simulink model "BLDCmotorControl_FOC_R2017b_fixdt"  (R2017b)
settings: Solver=FixedStepDiscrete  StartTime=0  StopTime=0.5  FixedStep=Ts  MaxStep=1e-6  RelTol=1e-6  AbsTol=1e-6  EnableMultiTasking=on
PreLoadFcn:
  | addpath(pwd);
  | addpath(genpath('01_Libraries'));
  | addpath(genpath('02_Figures'));
  | addpath(genpath('03_CreateParamTable'));
InitFcn:
  | init_model;
values from neighbouring files (symbols this model uses):
  a_elecAngle = 60    [init_model.m]
  b_diagEna = 1    [init_model.m]
  b_fieldWeakEna = 0    [init_model.m]
  b_selPhaABCurrMeas = 1    [init_model.m]
  cf_currFilt = 0.12    [init_model.m]
  cf_idKb = 1000 * Ts_ctrl    (= 0.06)    [init_model.m]
  cf_idKi = 100 * Ts_ctrl    (= 0.006)    [init_model.m]
  cf_idKp = 1    [init_model.m]
  cf_iqKb = 1000 * Ts_ctrl    (= 0.06)    [init_model.m]
  cf_iqKi = 100 * Ts_ctrl    (= 0.006)    [init_model.m]
  cf_iqKiLimProt = 40.7 * Ts_ctrl    (= 0.002442)    [init_model.m]
  cf_iqKp = 0.5    [init_model.m]
  cf_iqKpLimProt = 7.2    [init_model.m]
  cf_nKb = 1000 * Ts_ctrl    (= 0.06)    [init_model.m]
  cf_nKi = 20.4 * Ts_ctrl    (= 0.001224)    [init_model.m]
  cf_nKp = 1.18    [init_model.m]
  cf_nKpLimProt = 5    [init_model.m]
  cf_speedCoef = round(f_ctrl * a_mechAngle * (pi/180) * (30/pi))    [init_model.m]
  CTRL_COM = 0    [init_model.m]
  dV_openRate = 1000 * Ts_ctrl    (= 0.06)    [init_model.m]
  dz_cntTrnsDetHi = 40    [init_model.m]
  dz_cntTrnsDetLo = 20    [init_model.m]
  i_max = i_max * i_sca    (= 750)    [init_model.m]
  id_fieldWeak_M1 = [  0   0  0.05  0.25    1    2    3    4  4.5  4.8   5   5] * i_sca    [init_model.m]
  iq_max_M1 = sqrt(i_max^2 - iq_max_XA.^2)    [init_model.m]
  n_commAcvLo = 15    [init_model.m]
  n_commDeacvHi = 30    [init_model.m]
  n_max = 800    [init_model.m]
  n_stdStillDet = 3    [init_model.m]
  OPEN_MODE = 0    [init_model.m]
  r_cos_M1 = cos((a_elecAngle_XA + 30)*(pi/180))    [init_model.m]
  r_errInpTgtThres = 200    [init_model.m]
  r_sin_M1 = sin((a_elecAngle_XA + 30)*(pi/180))    [init_model.m]
  r_whl = 6.5 * 2.54 * 1e-2 / 2    (= 0.08255)    [init_model.m]
  SPD_MODE = 2    [init_model.m]
  t_errDequal = 2.0 * f_ctrl    (= 32000)    [init_model.m]
  t_errQual = 0.6 * f_ctrl    (= 9600)    [init_model.m]
  TRQ_MODE = 3    [init_model.m]
  Ts = 5e-6    (= 5e-06)    [init_model.m]
  Ts_ctrl = 6e-5    (= 6e-05)    [init_model.m]
  Vd_max = 1000 - V_margin    (= 900)    [init_model.m]
  vec_hallToPos = [0 2 0 1 4 3 5 0]    [init_model.m]
  VLT_MODE = 1    [init_model.m]
  Vq_max_M1 = sqrt(Vd_max^2 - Vq_max_XA.^2)    [init_model.m]
  z_commutMap_M1 = [-1 -1  0  1  1  0 ... (first row only)    [init_model.m]
  z_ctrlModReq = 1    [init_model.m]
  z_ctrlTypSel = 1    [init_model.m]
  z_maxCntRst = 2000    [init_model.m]
undefined symbols (not defined in the file or in its folder): DiscIntNeverNeededParam, sigbuilder_block, V_max, V_min
libraries: BLDC_controller_Lib x11, simulink x11, powerlib x6, pePwmGenerator x1
(part 2 of 3)

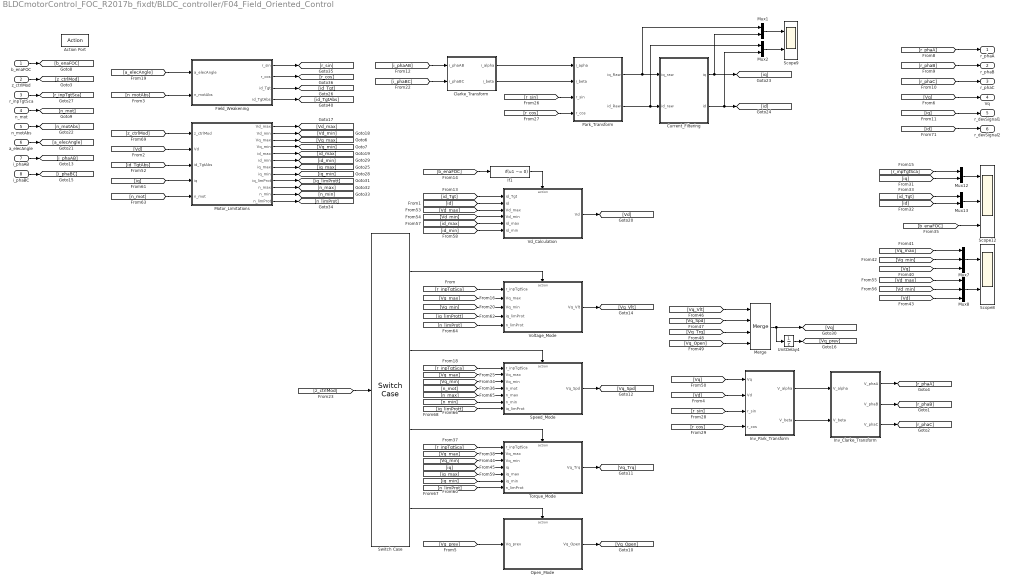
== system BLDCmotorControl_FOC_R2017b_fixdt/BLDC_controller/F04_Field_Oriented_Control ==
  b_enaFOC : Inport
  z_ctrlMod : Inport  Port=2
  r_inpTgtSca : Inport  Port=3
  n_mot : Inport  Port=4
  n_motAbs : Inport  Port=5
  a_elecAngle : Inport  Port=6
  i_phaAB : Inport  Port=7
  i_phaBC : Inport  Port=8
  Action Port : ActionPort  InitializeStates=reset  ActionType=then
  Clarke_Transform : Subsystem
  Current_Filtering : Subsystem
  Field_Weakening : Subsystem
  If1 : If  IfExpression=u1 ~= 0  ShowElse=off
  Inv_Clarke_Transform : Subsystem
  Inv_Park_Transform : Subsystem
  Merge : Merge  Inputs=4
  Motor_Limitations : Subsystem
  Mux{1..2,12..13} (4 alike) : Mux  Inputs=2
  Mux7 : Mux  Inputs=3
  Mux8 : Mux  Inputs=3
  Open_Mode : Subsystem
  Park_Transform : Subsystem
  Scope12 : Scope  NumInputPorts=3
  Scope8 : Scope  NumInputPorts=2
  Scope9 : Scope  NumInputPorts=2
  Speed_Mode : Subsystem
  Switch Case : SwitchCase  CaseConditions={VLT_MODE, SPD_MODE, TRQ_MODE}
  Torque_Mode : Subsystem
  UnitDelay4 : UnitDelay  SampleTime=-1
      settings: AttributesFormatString=Ini=%<X0>
  Vd_Calculation : Subsystem
  Voltage_Mode : Subsystem
  r_phaA : Outport  OutputWhenDisabled=reset  InitialOutput=0
  r_phaB : Outport  Port=2  OutputWhenDisabled=reset  InitialOutput=0
  "r_phaC " : Outport  Port=3  OutputWhenDisabled=reset  InitialOutput=0
  Vq : Outport  Port=4  OutputWhenDisabled=reset  InitialOutput=0
  r_devSignal1 : Outport  Port=5  OutputWhenDisabled=reset  InitialOutput=0
  r_devSignal2 : Outport  Port=6  OutputWhenDisabled=reset  InitialOutput=0
  wires:
  [r_phaA] -> r_phaA/1
  [r_phaB] -> r_phaB/1
  [r_phaC] -> "r_phaC "/1
  Inv_Park_Transform/1(V_alpha) -> Inv_Clarke_Transform/1(V_alpha)
  Inv_Park_Transform/2(V_beta) -> Inv_Clarke_Transform/2(V_beta)
  i_phaAB/1 -> [i_phaAB]
  i_phaBC/1 -> [i_phaBC]
  Inv_Clarke_Transform/1(V_phaA) -> [r_phaA]
  Inv_Clarke_Transform/2(V_phaB) -> [r_phaB]
  Inv_Clarke_Transform/3(V_phaC) -> [r_phaC]
  Clarke_Transform/1(i_alpha) -> Park_Transform/1(i_apha)
  Clarke_Transform/2(i_beta) -> Park_Transform/2(i_beta)
  Mux12/1 -> Scope12/1
  Mux13/1 -> Scope12/2
  [r_sin] -> Park_Transform/3(r_sin)
  [r_cos] -> Park_Transform/4(r_cos)
  [r_sin] -> Inv_Park_Transform/3(r_sin)
  [r_cos] -> Inv_Park_Transform/4(r_cos)
  [r_inpTgtSca] -> Mux12/1
  [iq] -> Mux12/2
  [id] -> Mux13/2
  [id_Tgt] -> Mux13/1
  r_inpTgtSca/1 -> [r_inpTgtSca]
  [i_phaAB] -> Clarke_Transform/1(i_phaAB)
  [i_phaBC] -> Clarke_Transform/2(i_phaBC)
  [Vd_max] -> Mux8/1
  [Vd] -> Mux8/3
  Mux8/1 -> Scope8/2
  [Vd_min] -> Mux8/2
  [Vq] -> Mux7/3
  Mux7/1 -> Scope8/1
  [Vq_max] -> Mux7/1
  [Vq_min] -> Mux7/2
  Park_Transform/2(id_Raw) -> Current_Filtering/2(id_raw), Mux2/1
  Park_Transform/1(iq_Raw) -> Current_Filtering/1(iq_raw), Mux1/1
  Current_Filtering/1(iq) -> [iq], Mux1/2
  Current_Filtering/2(id) -> [id], Mux2/2
  [Vq] -> Vq/1
  [id] -> Vd_Calculation/2(id)
  [id_Tgt] -> Vd_Calculation/1(id_Tgt)
  b_enaFOC/1 -> [b_enaFOC]
  If1/1 -> Vd_Calculation/Action
  [b_enaFOC] -> If1/1
  [Vd] -> Inv_Park_Transform/2(Vd)
  z_ctrlMod/1 -> [z_ctrlMod]
  n_mot/1 -> [n_mot]
  [b_enaFOC] -> Scope12/3
  [z_ctrlMod] -> Switch Case/1
  [Vq_prev] -> Open_Mode/1(Vq_prev)
  Open_Mode/1(Vq_Open) -> [Vq_Open]
  Torque_Mode/1(Vq_Trq) -> [Vq_Trq]
  Speed_Mode/1(Vq_Spd) -> [Vq_Spd]
  Voltage_Mode/1(Vq_Vlt) -> [Vq_Vlt]
  [r_inpTgtSca] -> Voltage_Mode/1(r_inpTgtSca)
  [Vq_max] -> Voltage_Mode/2(Vq_max)
  [Vq_min] -> Voltage_Mode/3(Vq_min)
  [r_inpTgtSca] -> Speed_Mode/1(r_inpTgtSca)
  [Vq_max] -> Speed_Mode/2(Vq_max)
  [Vq_min] -> Speed_Mode/3(Vq_min)
  [n_mot] -> Speed_Mode/4(n_mot)
  [Vq_min] -> Torque_Mode/3(Vq_min)
  [Vq_max] -> Torque_Mode/2(Vq_max)
  [r_inpTgtSca] -> Torque_Mode/1(r_inpTgtSca)
  [iq] -> Torque_Mode/4(iq)
  Switch Case/1 -> Voltage_Mode/Action
  Switch Case/2 -> Speed_Mode/Action
  Switch Case/3 -> Torque_Mode/Action
  Switch Case/4 -> Open_Mode/Action
  [Vq_Vlt] -> Merge/1
  [Vq_Spd] -> Merge/2
  [Vq_Trq] -> Merge/3
  [Vq_Open] -> Merge/4
  [Vq] -> Inv_Park_Transform/1(Vq)
  Merge/1 -> UnitDelay4/1, [Vq]
  UnitDelay4/1 -> [Vq_prev]
  Motor_Limitations/3(Vq_max) -> [Vq_max]
  Motor_Limitations/4(Vq_min) -> [Vq_min]
  [Vd] -> Motor_Limitations/2(Vd)
  [id_TgtAbs] -> Motor_Limitations/3(id_TgtAbs)
  Motor_Limitations/2(Vd_min) -> [Vd_min]
  Motor_Limitations/1(Vd_max) -> [Vd_max]
  [Vd_max] -> Vd_Calculation/3(Vd_max)
  [Vd_min] -> Vd_Calculation/4(Vd_min)
  Motor_Limitations/5(id_max) -> [id_max]
  Motor_Limitations/6(id_min) -> [id_min]
  Motor_Limitations/7(iq_max) -> [iq_max]
  Motor_Limitations/8(iq_min) -> [iq_min]
  [id_max] -> Vd_Calculation/5(id_max)
  [id_min] -> Vd_Calculation/6(id_min)
  [iq_max] -> Torque_Mode/5(iq_max)
  [iq_min] -> Torque_Mode/6(iq_min)
  [iq] -> Motor_Limitations/4(iq)
  Motor_Limitations/9(iq_limProt) -> [iq_limPrott]
  [iq_limPrott] -> Voltage_Mode/4(iq_limProt)
  Motor_Limitations/11(n_min) -> [n_min]
  Motor_Limitations/10(n_max) -> [n_max]
  Motor_Limitations/12(n_limProt) -> [n_limProt]
  [n_mot] -> Motor_Limitations/5(n_mot)
  [n_limProt] -> Voltage_Mode/5(n_limProt)
  [n_max] -> Speed_Mode/5(n_max)
  [n_min] -> Speed_Mode/6(n_min)
  [n_limProt] -> Torque_Mode/7(n_limProt)
  [iq_limPrott] -> Speed_Mode/7(iq_limProt)
  [z_ctrlMod] -> Motor_Limitations/1(z_ctrlMod)
  n_motAbs/1 -> [n_motAbs]
  Field_Weakening/1(r_sin) -> [r_sin]
  Field_Weakening/2(r_cos) -> [r_cos]
  [a_elecAngle] -> Field_Weakening/1(a_elecAngle)
  Field_Weakening/3(id_Tgt) -> [id_Tgt]
  [n_motAbs] -> Field_Weakening/2(n_motAbs)
  a_elecAngle/1 -> [a_elecAngle]
  Mux1/1 -> Scope9/1
  Mux2/1 -> Scope9/2
  [id] -> r_devSignal2/1
  [iq] -> r_devSignal1/1
  Field_Weakening/4(id_TgtAbs) -> [id_TgtAbs]
  Vd_Calculation/1(Vd) -> [Vd]

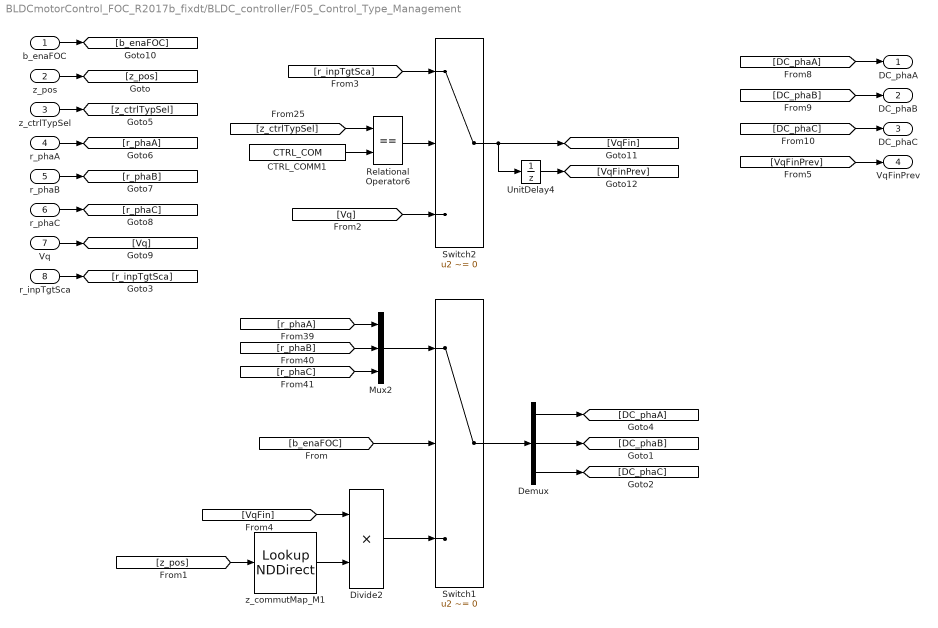
== system BLDCmotorControl_FOC_R2017b_fixdt/BLDC_controller/F05_Control_Type_Management ==
  b_enaFOC : Inport
  z_pos : Inport  Port=2
  z_ctrlTypSel : Inport  Port=3
  r_phaA : Inport  Port=4
  r_phaB : Inport  Port=5
  r_phaC : Inport  Port=6
  Vq : Inport  Port=7
  r_inpTgtSca : Inport  Port=8
  CTRL_COMM1 : Constant  Value=CTRL_COM  OutDataTypeStr=Inherit: Inherit via back propagation
  Demux : Demux  Outputs=3
  Divide2 : Product  Inputs=**  RndMeth=Simplest  OutDataTypeStr=Inherit: Same as first input
  Mux2 : Mux  Inputs=3
  Relational Operator6 : RelationalOperator  Operator===  OutDataTypeStr=boolean  RndMeth=Simplest
  Switch1 : Switch  Criteria=u2 ~= 0  OutDataTypeStr=Inherit: Inherit via back propagation  RndMeth=Zero
  Switch2 : Switch  Criteria=u2 ~= 0  OutDataTypeStr=Inherit: Inherit via back propagation  RndMeth=Zero
  UnitDelay4 : UnitDelay  SampleTime=-1
      settings: AttributesFormatString=Ini=%<X0>
  z_commutMap_M1 : LookupNDDirect  InputsSelectThisObjectFromTable=Column  Table=z_commutMap_M1  DiagnosticForOutOfRangeInput=None  TableDataTypeStr=int16
  DC_phaA : Outport  OutputWhenDisabled=reset  InitialOutput=0
  DC_phaB : Outport  Port=2  OutputWhenDisabled=reset  InitialOutput=0
  "DC_phaC " : Outport  Port=3  OutputWhenDisabled=reset  InitialOutput=0
  VqFinPrev : Outport  Port=4  OutputWhenDisabled=reset  InitialOutput=0
  wires:
  Demux/3 -> [DC_phaC]
  Demux/2 -> [DC_phaB]
  Demux/1 -> [DC_phaA]
  z_pos/1 -> [z_pos]
  [DC_phaC] -> "DC_phaC "/1
  [DC_phaB] -> DC_phaB/1
  [DC_phaA] -> DC_phaA/1
  [z_pos] -> z_commutMap_M1/1
  Switch1/1 -> Demux/1
  r_phaA/1 -> [r_phaA]
  r_phaB/1 -> [r_phaB]
  r_phaC/1 -> [r_phaC]
  Vq/1 -> [Vq]
  [r_phaA] -> Mux2/1
  [r_phaB] -> Mux2/2
  [r_phaC] -> Mux2/3
  z_commutMap_M1/1 -> Divide2/2
  Divide2/1 -> Switch1/3
  b_enaFOC/1 -> [b_enaFOC]
  Mux2/1 -> Switch1/1
  [b_enaFOC] -> Switch1/2
  [z_ctrlTypSel] -> Relational Operator6/1
  CTRL_COMM1/1 -> Relational Operator6/2
  Relational Operator6/1 -> Switch2/2
  r_inpTgtSca/1 -> [r_inpTgtSca]
  [Vq] -> Switch2/3
  z_ctrlTypSel/1 -> [z_ctrlTypSel]
  Switch2/1 -> UnitDelay4/1, [VqFin]
  UnitDelay4/1 -> [VqFinPrev]
  [VqFin] -> Divide2/1
  [VqFinPrev] -> VqFinPrev/1
  [r_inpTgtSca] -> Switch2/1

== system BLDCmotorControl_FOC_R2017b_fixdt/BLDC_controller/Implemented_control_methods ==

== system BLDCmotorControl_FOC_R2017b_fixdt/BLDC_model_closed/__InputSSForSFun__ ==
  gates_PWM : Inport
  Tm_Nm : Inport  Port=2
  __UniqueOutportName__1__ : Outport
  __UniqueOutportName__2__ : Outport  Port=2
  wires:
  gates_PWM/1 -> __UniqueOutportName__1__/1
  Tm_Nm/1 -> __UniqueOutportName__2__/1

== system BLDCmotorControl_FOC_R2017b_fixdt/BLDC_model_closed/__OutputSSForSFun__ ==
  __UniqueInportName__1__ : Inport
  __UniqueInportName__2__ : Inport  Port=2
  __UniqueInportName__3__ : Inport  Port=3
  __UniqueInportName__4__ : Inport  Port=4
  __UniqueInportName__5__ : Inport  Port=5
  __UniqueInportName__6__ : Inport  Port=6
  __UniqueInportName__7__ : Inport  Port=7
  __UniqueInportName__8__ : Inport  Port=8
  __UniqueInportName__9__ : Inport  Port=9
  __UniqueInportName__10__ : Inport  Port=10
  __UniqueInportName__11__ : Inport  Port=11
  __UniqueInportName__12__ : Inport  Port=12
  Mux1 : BusCreator  Inputs=12
  motor_out : Outport
  wires:
  __UniqueInportName__1__/1 -> Mux1/1  "Stator current is_a (A)"
  __UniqueInportName__2__/1 -> Mux1/2  "Stator current is_b (A)"
  __UniqueInportName__3__/1 -> Mux1/3  "Stator current is_c (A)"
  __UniqueInportName__4__/1 -> Mux1/4  "Stator back EMF e_a (V)"
  __UniqueInportName__5__/1 -> Mux1/5  "Stator back EMF e_b (V)"
  __UniqueInportName__6__/1 -> Mux1/6  "Stator back EMF e_cV)"
  __UniqueInportName__7__/1 -> Mux1/7  "Hall effect signal h_a"
  __UniqueInportName__8__/1 -> Mux1/8  "Hall effect signal h_b"
  __UniqueInportName__9__/1 -> Mux1/9  "Hall effect signal h_c"
  __UniqueInportName__10__/1 -> Mux1/10  "Rotor speed wm (rad/s)"
  __UniqueInportName__11__/1 -> Mux1/11  "Rotor angle thetam (rad)"
  __UniqueInportName__12__/1 -> Mux1/12  "Electromagnetic torque Te (N*m)"
  Mux1/1 -> motor_out/1

== system BLDCmotorControl_FOC_R2017b_fixdt/PWM_gates/PWM_generator1 ==
  DC : Inport  SampleTime=Ts
  PWM_generator_sfcn : S-Function  FunctionName=PWM_generator_sf  SFunctionModules=""  SFunctionDeploymentMode=off  EnableBusSupport=off  SFcnStateName=DWORK0  mask{rtw_sf_name=PWM_generator_sf, showVar=off}
      mask prompts: rtw_sf_name "Simulink:masks:GenSFuncName_MP"; showVar "Simulink:masks:GenSFuncShowModuleList_MP"
      mask help: Simulink:masks:GenSFuncDesc_MD
      mask init: same as BLDCmotorControl_FOC_R2017b_fixdt/BLDC_model_closed/BLDC_model_sfcn
      settings: SFcnIsStateOwnerBlock=on
      settings: CopyFcn=|
      | if ~strcmp(get_param(gcb,'Linkstatus'),'none') && ...
      | ~strcmp(get_param(gcb,'Linkstatus'),'implicit')
      |   set_param(gcb,'LinkStatus','none');
      | end
      mask Help: eval('feval(''rtwprivate'',''rtwhelpview'',''rtw_sfcn_block'')');
      mask Display:
      | port_label('input',1,'DC');
      | port_label('output',1,'PWM');
  __InputSSForSFun__ : Subsystem
  __OutputSSForSFun__ : Subsystem
  PWM : Outport
  wires:
  __OutputSSForSFun__/1(PWM) -> PWM/1
  PWM_generator_sfcn/1 -> __OutputSSForSFun__/1(__UniqueInportName__1__)
  __InputSSForSFun__/1(__UniqueOutportName__1__) -> PWM_generator_sfcn/1
  DC/1 -> __InputSSForSFun__/1(DC)

== system BLDCmotorControl_FOC_R2017b_fixdt/PWM_gates/PWM_generator12 ==
  DC : Inport  SampleTime=Ts
  PWM_generator_sfcn : S-Function  FunctionName=PWM_generator_sf  SFunctionModules=""  SFunctionDeploymentMode=off  EnableBusSupport=off  SFcnStateName=DWORK0  mask{rtw_sf_name=PWM_generator_sf, showVar=off}
      mask prompts: rtw_sf_name "Simulink:masks:GenSFuncName_MP"; showVar "Simulink:masks:GenSFuncShowModuleList_MP"
      mask help: Simulink:masks:GenSFuncDesc_MD
      mask init: same as BLDCmotorControl_FOC_R2017b_fixdt/BLDC_model_closed/BLDC_model_sfcn
      settings: SFcnIsStateOwnerBlock=on
      settings: CopyFcn=|
      | if ~strcmp(get_param(gcb,'Linkstatus'),'none') && ...
      | ~strcmp(get_param(gcb,'Linkstatus'),'implicit')
      |   set_param(gcb,'LinkStatus','none');
      | end
      mask Help: eval('feval(''rtwprivate'',''rtwhelpview'',''rtw_sfcn_block'')');
      mask Display:
      | port_label('input',1,'DC');
      | port_label('output',1,'PWM');
  __InputSSForSFun__ : Subsystem
  __OutputSSForSFun__ : Subsystem
  PWM : Outport
  wires:
  DC/1 -> __InputSSForSFun__/1(DC)
  __InputSSForSFun__/1(__UniqueOutportName__1__) -> PWM_generator_sfcn/1
  PWM_generator_sfcn/1 -> __OutputSSForSFun__/1(__UniqueInportName__1__)
  __OutputSSForSFun__/1(PWM) -> PWM/1

== system BLDCmotorControl_FOC_R2017b_fixdt/PWM_gates/PWM_generator2 ==
  DC : Inport  SampleTime=Ts
  PWM_generator_sfcn : S-Function  FunctionName=PWM_generator_sf  SFunctionModules=""  SFunctionDeploymentMode=off  EnableBusSupport=off  SFcnStateName=DWORK0  mask{rtw_sf_name=PWM_generator_sf, showVar=off}
      mask prompts: rtw_sf_name "Simulink:masks:GenSFuncName_MP"; showVar "Simulink:masks:GenSFuncShowModuleList_MP"
      mask help: Simulink:masks:GenSFuncDesc_MD
      mask init: same as BLDCmotorControl_FOC_R2017b_fixdt/BLDC_model_closed/BLDC_model_sfcn
      settings: SFcnIsStateOwnerBlock=on
      settings: CopyFcn=|
      | if ~strcmp(get_param(gcb,'Linkstatus'),'none') && ...
      | ~strcmp(get_param(gcb,'Linkstatus'),'implicit')
      |   set_param(gcb,'LinkStatus','none');
      | end
      mask Help: eval('feval(''rtwprivate'',''rtwhelpview'',''rtw_sfcn_block'')');
      mask Display:
      | port_label('input',1,'DC');
      | port_label('output',1,'PWM');
  __InputSSForSFun__ : Subsystem
  __OutputSSForSFun__ : Subsystem
  PWM : Outport
  wires:
  DC/1 -> __InputSSForSFun__/1(DC)
  __InputSSForSFun__/1(__UniqueOutportName__1__) -> PWM_generator_sfcn/1
  PWM_generator_sfcn/1 -> __OutputSSForSFun__/1(__UniqueInportName__1__)
  __OutputSSForSFun__/1(PWM) -> PWM/1

== system BLDCmotorControl_FOC_R2017b_fixdt/PWM_gates/PWM_generator3 ==
  DC : Inport  SampleTime=Ts
  PWM_generator_sfcn : S-Function  FunctionName=PWM_generator_sf  SFunctionModules=""  SFunctionDeploymentMode=off  EnableBusSupport=off  SFcnStateName=DWORK0  mask{rtw_sf_name=PWM_generator_sf, showVar=off}
      mask prompts: rtw_sf_name "Simulink:masks:GenSFuncName_MP"; showVar "Simulink:masks:GenSFuncShowModuleList_MP"
      mask help: Simulink:masks:GenSFuncDesc_MD
      mask init: same as BLDCmotorControl_FOC_R2017b_fixdt/BLDC_model_closed/BLDC_model_sfcn
      settings: SFcnIsStateOwnerBlock=on
      settings: CopyFcn=|
      | if ~strcmp(get_param(gcb,'Linkstatus'),'none') && ...
      | ~strcmp(get_param(gcb,'Linkstatus'),'implicit')
      |   set_param(gcb,'LinkStatus','none');
      | end
      mask Help: eval('feval(''rtwprivate'',''rtwhelpview'',''rtw_sfcn_block'')');
      mask Display:
      | port_label('input',1,'DC');
      | port_label('output',1,'PWM');
  __InputSSForSFun__ : Subsystem
  __OutputSSForSFun__ : Subsystem
  PWM : Outport
  wires:
  __OutputSSForSFun__/1(PWM) -> PWM/1
  PWM_generator_sfcn/1 -> __OutputSSForSFun__/1(__UniqueInportName__1__)
  __InputSSForSFun__/1(__UniqueOutportName__1__) -> PWM_generator_sfcn/1
  DC/1 -> __InputSSForSFun__/1(DC)

== system BLDCmotorControl_FOC_R2017b_fixdt/PWM_gates/PWM_generator4 ==
  DC : Inport  SampleTime=Ts
  PWM_generator_sfcn : S-Function  FunctionName=PWM_generator_sf  SFunctionModules=""  SFunctionDeploymentMode=off  EnableBusSupport=off  SFcnStateName=DWORK0  mask{rtw_sf_name=PWM_generator_sf, showVar=off}
      mask prompts: rtw_sf_name "Simulink:masks:GenSFuncName_MP"; showVar "Simulink:masks:GenSFuncShowModuleList_MP"
      mask help: Simulink:masks:GenSFuncDesc_MD
      mask init: same as BLDCmotorControl_FOC_R2017b_fixdt/BLDC_model_closed/BLDC_model_sfcn
      settings: SFcnIsStateOwnerBlock=on
      settings: CopyFcn=|
      | if ~strcmp(get_param(gcb,'Linkstatus'),'none') && ...
      | ~strcmp(get_param(gcb,'Linkstatus'),'implicit')
      |   set_param(gcb,'LinkStatus','none');
      | end
      mask Help: eval('feval(''rtwprivate'',''rtwhelpview'',''rtw_sfcn_block'')');
      mask Display:
      | port_label('input',1,'DC');
      | port_label('output',1,'PWM');
  __InputSSForSFun__ : Subsystem
  __OutputSSForSFun__ : Subsystem
  PWM : Outport
  wires:
  DC/1 -> __InputSSForSFun__/1(DC)
  __InputSSForSFun__/1(__UniqueOutportName__1__) -> PWM_generator_sfcn/1
  PWM_generator_sfcn/1 -> __OutputSSForSFun__/1(__UniqueInportName__1__)
  __OutputSSForSFun__/1(PWM) -> PWM/1

== system BLDCmotorControl_FOC_R2017b_fixdt/PWM_gates/PWM_generator5 ==
  DC : Inport  SampleTime=Ts
  PWM_generator_sfcn : S-Function  FunctionName=PWM_generator_sf  SFunctionModules=""  SFunctionDeploymentMode=off  EnableBusSupport=off  SFcnStateName=DWORK0  mask{rtw_sf_name=PWM_generator_sf, showVar=off}
      mask prompts: rtw_sf_name "Simulink:masks:GenSFuncName_MP"; showVar "Simulink:masks:GenSFuncShowModuleList_MP"
      mask help: Simulink:masks:GenSFuncDesc_MD
      mask init: same as BLDCmotorControl_FOC_R2017b_fixdt/BLDC_model_closed/BLDC_model_sfcn
      settings: SFcnIsStateOwnerBlock=on
      settings: CopyFcn=|
      | if ~strcmp(get_param(gcb,'Linkstatus'),'none') && ...
      | ~strcmp(get_param(gcb,'Linkstatus'),'implicit')
      |   set_param(gcb,'LinkStatus','none');
      | end
      mask Help: eval('feval(''rtwprivate'',''rtwhelpview'',''rtw_sfcn_block'')');
      mask Display:
      | port_label('input',1,'DC');
      | port_label('output',1,'PWM');
  __InputSSForSFun__ : Subsystem
  __OutputSSForSFun__ : Subsystem
  PWM : Outport
  wires:
  __OutputSSForSFun__/1(PWM) -> PWM/1
  PWM_generator_sfcn/1 -> __OutputSSForSFun__/1(__UniqueInportName__1__)
  __InputSSForSFun__/1(__UniqueOutportName__1__) -> PWM_generator_sfcn/1
  DC/1 -> __InputSSForSFun__/1(DC)

== system BLDCmotorControl_FOC_R2017b_fixdt/PWM_gates/signal_log6 ==
  PWM : Inport
  Terminator_1 : Terminator
  wires:
  PWM/1 -> Terminator_1/1  "PWM"

== system BLDCmotorControl_FOC_R2017b_fixdt/filtLowPass/Low_Pass_Filter1 ==
  u : Inport
  coef : Inport  Port=2
  Constant1 : Constant  OutDataTypeStr=Inherit: Inherit via back propagation
  Divide1 : Product  Inputs=**  RndMeth=Simplest  OutDataTypeStr=Inherit: Same as first input
  Divide2 : Product  Inputs=**  RndMeth=Simplest  OutDataTypeStr=Inherit: Same as first input
  Sum1 : Sum  OutDataTypeStr=fixdt(1,16,4)  RndMeth=Simplest  SaturateOnIntegerOverflow=on  InputSameDT=on
  Sum5 : Sum  Inputs=+-  RndMeth=Simplest  InputSameDT=on  OutDataTypeStr=Inherit: Same as first input
  UnitDelay3 : UnitDelay  SampleTime=-1
  y : Outport
  wires:
  u/1 -> Divide1/1
  Sum1/1 -> UnitDelay3/1, y/1
  Constant1/1 -> Sum5/1
  Divide2/1 -> Sum1/2
  UnitDelay3/1 -> Divide2/1
  Sum5/1 -> Divide2/2
  coef/1 -> Sum5/2, Divide1/2
  Divide1/1 -> Sum1/1

== system BLDCmotorControl_FOC_R2017b_fixdt/BLDC_controller/F01_Estimations/F01_01_Input_Scaling ==
  note: Input Scaling [-1000,1000] → [min,max]
  z_ctrlTypSel : Inport
  r_inpTgt : Inport  Port=2
  z_ctrlModPrev : Inport  Port=3
  Commutation_Control_Type : Subsystem
  FOC_Control_Type : Subsystem
  If1 : If  IfExpression=u1 == CTRL_COM
  Merge : Merge
  r_inpTgtSca : Outport  OutputWhenDisabled=reset  InitialOutput=0
  wires:
  Commutation_Control_Type/1(r_inpTgtScaCOM) -> Merge/1
  [r_inpTgt] -> FOC_Control_Type/1(r_inpTgt)
  [r_inpTgtSca] -> r_inpTgtSca/1
  If1/1 -> Commutation_Control_Type/Action
  z_ctrlTypSel/1 -> [z_ctrlTypSel]
  [z_ctrlTypSel] -> If1/1
  FOC_Control_Type/1(r_inpTgtScaFOC) -> Merge/2
  [r_inpTgt] -> Commutation_Control_Type/1(r_inpTgt)
  r_inpTgt/1 -> [r_inpTgt]
  Merge/1 -> [r_inpTgtSca]
  If1/2 -> FOC_Control_Type/Action
  [z_ctrlModPrev] -> FOC_Control_Type/2(z_ctrlModPrev)
  z_ctrlModPrev/1 -> [z_ctrlModPrev]

== system BLDCmotorControl_FOC_R2017b_fixdt/BLDC_controller/F01_Estimations/F01_02_Edge_Detector ==
  b_hallA : Inport
  b_hallB : Inport  Port=2
  b_hallC : Inport  Port=3
  Logical Operator : Logic  Operator=XOR  Inputs=6  AllPortsSameDT=off  OutDataTypeStr=boolean
  UnitDelay1 : UnitDelay  SampleTime=-1
      settings: AttributesFormatString=Ini=%<X0>
  UnitDelay2 : UnitDelay  SampleTime=-1
      settings: AttributesFormatString=Ini=%<X0>
  UnitDelay3 : UnitDelay  SampleTime=-1
      settings: AttributesFormatString=Ini=%<X0>
  "b_edge " : Outport  OutputWhenDisabled=reset  InitialOutput=0
  wires:
  b_hallA/1 -> Logical Operator/1, UnitDelay3/1
  b_hallC/1 -> Logical Operator/3, UnitDelay2/1
  b_hallB/1 -> Logical Operator/2, UnitDelay1/1
  UnitDelay1/1 -> Logical Operator/5
  UnitDelay2/1 -> Logical Operator/6
  UnitDelay3/1 -> Logical Operator/4
  Logical Operator/1 -> "b_edge "/1

== system BLDCmotorControl_FOC_R2017b_fixdt/BLDC_controller/F01_Estimations/F01_03_Position_Calculation ==
  note: This calculates the low resolution position based on Hall sensors.
  b_hallA : Inport
  b_hallB : Inport  Port=2
  b_hallC : Inport  Port=3
  Selector : Selector  IndexMode=Zero-based  InputPortWidth=length(vec_hallToPos)  IndexOptions=Index vector (port)  Indices=[1 3]  OutputSizes=1
  Sum : Sum  Inputs=+++  RndMeth=Simplest  OutDataTypeStr=Inherit: Same as first input
  g_Ha : Gain  Gain=4  OutDataTypeStr=Inherit: Inherit via back propagation  RndMeth=Zero  ParamDataTypeStr=Inherit: Same as input
  g_Hb : Gain  Gain=2  OutDataTypeStr=Inherit: Inherit via back propagation  RndMeth=Simplest  ParamDataTypeStr=Inherit: Same as input
  vec_hallToPos : Constant  Value=vec_hallToPos  OutDataTypeStr=int8
  z_posRaw : Outport  OutputWhenDisabled=reset  InitialOutput=0
  "z_pos " : Outport  Port=2  OutputWhenDisabled=reset  InitialOutput=0
  wires:
  b_hallC/1 -> Sum/3
  g_Ha/1 -> Sum/1
  g_Hb/1 -> Sum/2
  Sum/1 -> z_posRaw/1, Selector/2
  b_hallA/1 -> g_Ha/1
  b_hallB/1 -> g_Hb/1
  vec_hallToPos/1 -> Selector/1
  Selector/1 -> "z_pos "/1

== system BLDCmotorControl_FOC_R2017b_fixdt/BLDC_controller/F01_Estimations/F01_04_Direction_Detection ==
  z_pos : Inport
  Action Port : ActionPort  ActionType=then
  Constant20 : Constant  Value=-5  OutDataTypeStr=Inherit: Inherit via back propagation
  Constant23 : Constant  Value=-1  OutDataTypeStr=int8
  Constant24 : Constant  OutDataTypeStr=int8
  Constant8 : Constant  OutDataTypeStr=Inherit: Inherit via back propagation
  Logical Operator3 : Logic  Operator=OR  AllPortsSameDT=off  OutDataTypeStr=boolean
  Relational Operator1 : RelationalOperator  Operator===  OutDataTypeStr=boolean  RndMeth=Simplest
  Relational Operator6 : RelationalOperator  Operator===  OutDataTypeStr=boolean  RndMeth=Simplest
  Sum2 : Sum  Inputs=|+-  RndMeth=Zero  InputSameDT=on  OutDataTypeStr=Inherit: Same as first input
  Switch2 : Switch  Criteria=u2 ~= 0  OutDataTypeStr=Inherit: Inherit via back propagation  RndMeth=Simplest
  UnitDelay2 : UnitDelay  SampleTime=-1
  UnitDelay3 : UnitDelay  SampleTime=-1
      settings: AttributesFormatString=Ini=%<X0>
  z_dir : Outport
  z_dirPrev : Outport  Port=2
  wires:
  UnitDelay2/1 -> Sum2/2
  Relational Operator1/1 -> Logical Operator3/1
  Constant8/1 -> Relational Operator1/2
  Sum2/1 -> Relational Operator6/1, Relational Operator1/1
  Relational Operator6/1 -> Logical Operator3/2
  Constant20/1 -> Relational Operator6/2
  Constant24/1 -> Switch2/1
  Constant23/1 -> Switch2/3
  Logical Operator3/1 -> Switch2/2
  z_pos/1 -> Sum2/1, UnitDelay2/1
  Switch2/1 -> UnitDelay3/1, z_dir/1
  UnitDelay3/1 -> z_dirPrev/1

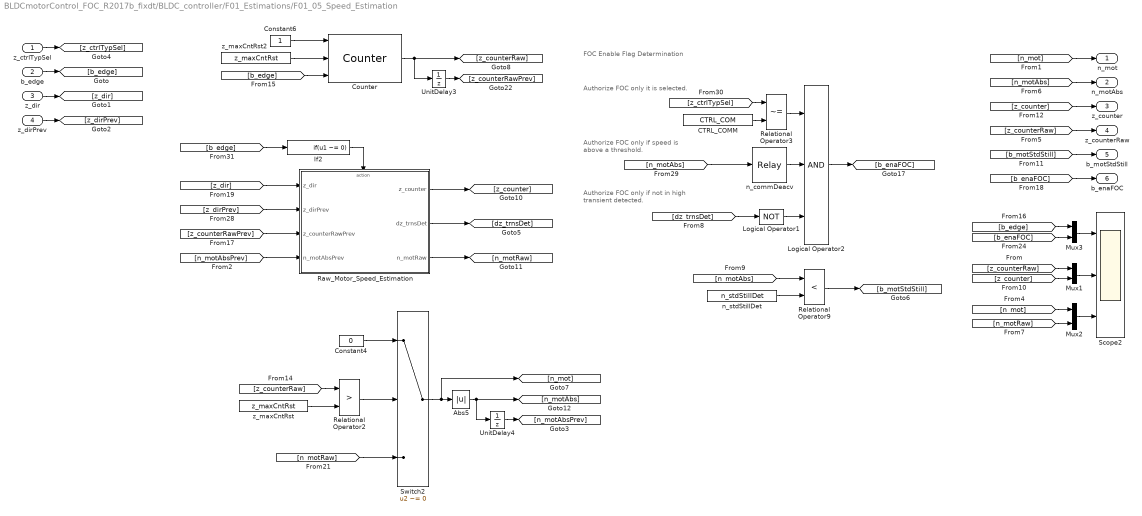
== system BLDCmotorControl_FOC_R2017b_fixdt/BLDC_controller/F01_Estimations/F01_05_Speed_Estimation ==
  note: FOC Enable Flag Determination
  note: Authorize FOC only if speed is above a threshold.
  note: Authorize FOC only if not in high transient detected.
  note: Authorize FOC only it is selected.
  z_ctrlTypSel : Inport
  b_edge : Inport  Port=2
  z_dir : Inport  Port=3
  z_dirPrev : Inport  Port=4
  Abs5 : Abs  OutDataTypeStr=Inherit: Inherit via back propagation  RndMeth=Zero
  CTRL_COMM : Constant  Value=CTRL_COM  OutDataTypeStr=Inherit: Inherit via back propagation
  Constant4 : Constant  Value=0  OutDataTypeStr=Inherit: Inherit via back propagation
  Constant6 : Constant  OutDataTypeStr=fixdt(1,16,0)
  Counter : BLDC_controller_Lib/Counter  z_cntInit=z_maxCntRst
      settings: AttributesFormatString=Ini=%<z_cntInit>
  If2 : If  IfExpression=u1 ~= 0  ShowElse=off
  Logical Operator1 : Logic  Operator=NOT  AllPortsSameDT=off  OutDataTypeStr=boolean
  Logical Operator2 : Logic  Inputs=3  AllPortsSameDT=off  OutDataTypeStr=boolean
  Mux1 : Mux  Inputs=2
  Mux2 : Mux  Inputs=2
  Mux3 : Mux  Inputs=2
  Raw_Motor_Speed_Estimation : Subsystem
  Relational Operator2 : RelationalOperator  Operator=>  OutDataTypeStr=boolean  RndMeth=Simplest
  Relational Operator3 : RelationalOperator  Operator=~=  OutDataTypeStr=boolean  RndMeth=Simplest
  Relational Operator9 : RelationalOperator  Operator=<  OutDataTypeStr=boolean  RndMeth=Simplest
  Scope2 : Scope  NumInputPorts=3
  Switch2 : Switch  Criteria=u2 ~= 0  OutDataTypeStr=Inherit: Inherit via back propagation  RndMeth=Zero
  UnitDelay3 : UnitDelay  InitialCondition=z_maxCntRst  SampleTime=-1
      settings: AttributesFormatString=Ini=%<X0>
  UnitDelay4 : UnitDelay  SampleTime=-1
      settings: AttributesFormatString=Ini=%<X0>
  n_commDeacv : Relay  OnSwitchValue=n_commDeacvHi  OffSwitchValue=n_commAcvLo  OutDataTypeStr=boolean
  n_stdStillDet : Constant  Value=n_stdStillDet  OutDataTypeStr=Inherit: Inherit via back propagation
  z_maxCntRst : Constant  Value=z_maxCntRst  OutDataTypeStr=Inherit: Inherit via back propagation
  z_maxCntRst2 : Constant  Value=z_maxCntRst  OutDataTypeStr=Inherit: Inherit via back propagation
  n_mot : Outport
  n_motAbs : Outport  Port=2
  z_counter : Outport  Port=3  OutputWhenDisabled=reset  InitialOutput=0
  z_counterRaw : Outport  Port=4  OutputWhenDisabled=reset  InitialOutput=0
  b_motStdStill : Outport  Port=5  OutputWhenDisabled=reset  InitialOutput=0
  b_enaFOC : Outport  Port=6
  wires:
  [n_motRaw] -> Mux2/2
  Mux2/1 -> Scope2/3
  [n_mot] -> Mux2/1
  Mux1/1 -> Scope2/2
  [z_counterRaw] -> Mux1/1
  [z_counter] -> Mux1/2
  b_edge/1 -> [b_edge]
  [n_mot] -> n_mot/1
  z_dir/1 -> [z_dir]
  [z_counter] -> z_counter/1
  [z_counterRaw] -> z_counterRaw/1
  UnitDelay3/1 -> [z_counterRawPrev]
  z_dirPrev/1 -> [z_dirPrev]
  [z_dir] -> Raw_Motor_Speed_Estimation/1(z_dir)
  Abs5/1 -> UnitDelay4/1, [n_motAbs]
  Raw_Motor_Speed_Estimation/1(z_counter) -> [z_counter]
  [z_dirPrev] -> Raw_Motor_Speed_Estimation/2(z_dirPrev)
  If2/1 -> Raw_Motor_Speed_Estimation/Action
  [z_counterRawPrev] -> Raw_Motor_Speed_Estimation/3(z_counterRawPrev)
  [b_enaFOC] -> b_enaFOC/1
  z_ctrlTypSel/1 -> [z_ctrlTypSel]
  [z_counterRaw] -> Relational Operator2/1
  z_maxCntRst/1 -> Relational Operator2/2
  Constant4/1 -> Switch2/1
  Raw_Motor_Speed_Estimation/3(n_motRaw) -> [n_motRaw]
  Switch2/1 -> [n_mot], Abs5/1
  Mux3/1 -> Scope2/1
  [b_enaFOC] -> Mux3/2
  [b_edge] -> Mux3/1
  [b_edge] -> If2/1
  Relational Operator2/1 -> Switch2/2
  UnitDelay4/1 -> [n_motAbsPrev]
  [n_motAbsPrev] -> Raw_Motor_Speed_Estimation/4(n_motAbsPrev)
  [n_motAbs] -> n_motAbs/1
  CTRL_COMM/1 -> Relational Operator3/2
  [z_ctrlTypSel] -> Relational Operator3/1
  [n_motAbs] -> n_commDeacv/1
  Raw_Motor_Speed_Estimation/2(dz_trnsDet) -> [dz_trnsDet]
  Relational Operator3/1 -> Logical Operator2/1
  n_commDeacv/1 -> Logical Operator2/2
  Logical Operator1/1 -> Logical Operator2/3
  Logical Operator2/1 -> [b_enaFOC]
  [dz_trnsDet] -> Logical Operator1/1
  z_maxCntRst2/1 -> Counter/2
  [b_edge] -> Counter/3
  Constant6/1 -> Counter/1
  Counter/1 -> UnitDelay3/1, [z_counterRaw]
  [b_motStdStill] -> b_motStdStill/1
  [n_motAbs] -> Relational Operator9/1
  n_stdStillDet/1 -> Relational Operator9/2
  Relational Operator9/1 -> [b_motStdStill]
  [n_motRaw] -> Switch2/3

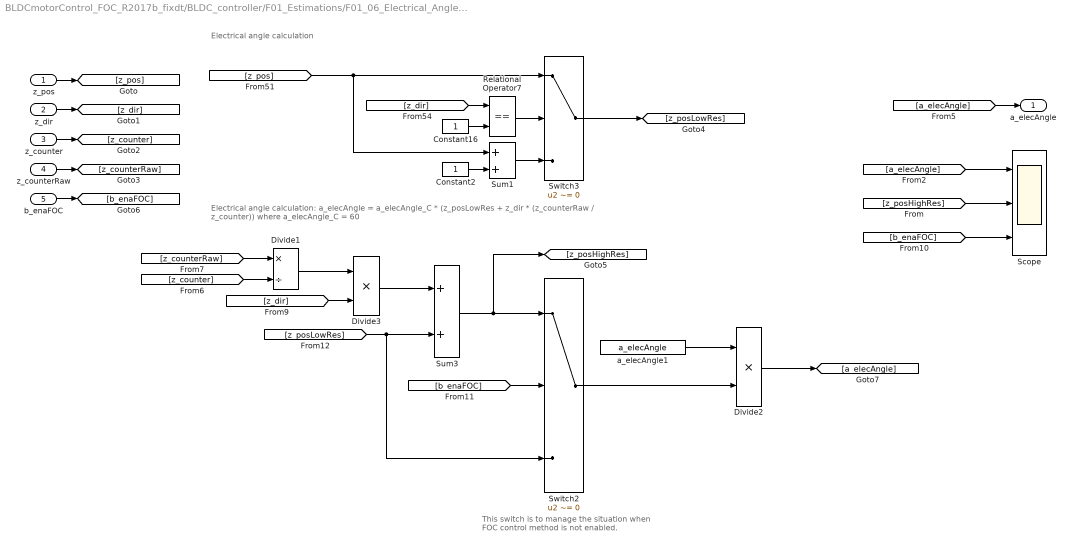
== system BLDCmotorControl_FOC_R2017b_fixdt/BLDC_controller/F01_Estimations/F01_06_Electrical_Angle_Estimation ==
  note: Electrical angle calculation
  note: This switch is to manage the situation when FOC control method is not enabled.
  note: Electrical angle calculation:
      | a_elecAngle = a_elecAngle_C * (z_posLowRes + z_dir * (z_counterRaw / z_counter))
      | where a_elecAngle_C = 60
  z_pos : Inport
  z_dir : Inport  Port=2
  z_counter : Inport  Port=3
  z_counterRaw : Inport  Port=4
  b_enaFOC : Inport  Port=5
  Constant16 : Constant  OutDataTypeStr=Inherit: Inherit via back propagation
  Constant2 : Constant  OutDataTypeStr=Inherit: Inherit via back propagation
  Divide1 : Product  Inputs=*/  OutDataTypeStr=fixdt(0,16,16)  RndMeth=Simplest  SaturateOnIntegerOverflow=on
  Divide2 : Product  Inputs=**  RndMeth=Simplest  OutDataTypeStr=Inherit: Same as first input
  Divide3 : Product  Inputs=**  OutDataTypeStr=fixdt(1,16,15)  RndMeth=Simplest
  Relational Operator7 : RelationalOperator  Operator===  OutDataTypeStr=boolean  RndMeth=Simplest
  Scope : Scope  NumInputPorts=3
  Sum1 : Sum  RndMeth=Simplest  OutDataTypeStr=Inherit: Same as first input
  Sum3 : Sum  OutDataTypeStr=fixdt(0,16,12)  RndMeth=Simplest
  Switch2 : Switch  Criteria=u2 ~= 0  OutDataTypeStr=Inherit: Inherit via back propagation  RndMeth=Zero
  Switch3 : Switch  Criteria=u2 ~= 0  OutDataTypeStr=Inherit: Inherit via back propagation  RndMeth=Zero
  a_elecAngle1 : Constant  Value=a_elecAngle  OutDataTypeStr=fixdt(0,16,6)
  a_elecAngle : Outport  OutputWhenDisabled=reset  InitialOutput=0
  wires:
  z_pos/1 -> [z_pos]
  z_dir/1 -> [z_dir]
  [a_elecAngle] -> Scope/1
  [b_enaFOC] -> Scope/3
  z_counterRaw/1 -> [z_counterRaw]
  z_counter/1 -> [z_counter]
  [z_pos] -> Switch3/1, Sum1/1
  Constant2/1 -> Sum1/2
  Relational Operator7/1 -> Switch3/2
  Constant16/1 -> Relational Operator7/2
  [z_dir] -> Relational Operator7/1
  Sum1/1 -> Switch3/3
  b_enaFOC/1 -> [b_enaFOC]
  [a_elecAngle] -> a_elecAngle/1
  [z_counterRaw] -> Divide1/1
  [z_counter] -> Divide1/2
  a_elecAngle1/1 -> Divide2/1
  [b_enaFOC] -> Switch2/2
  Switch2/1 -> Divide2/2
  Sum3/1 -> [z_posHighRes], Switch2/1
  Divide3/1 -> Sum3/1
  Divide2/1 -> [a_elecAngle]
  [z_posLowRes] -> Switch2/3, Sum3/2
  Switch3/1 -> [z_posLowRes]
  [z_posHighRes] -> Scope/2
  Divide1/1 -> Divide3/1
  [z_dir] -> Divide3/2

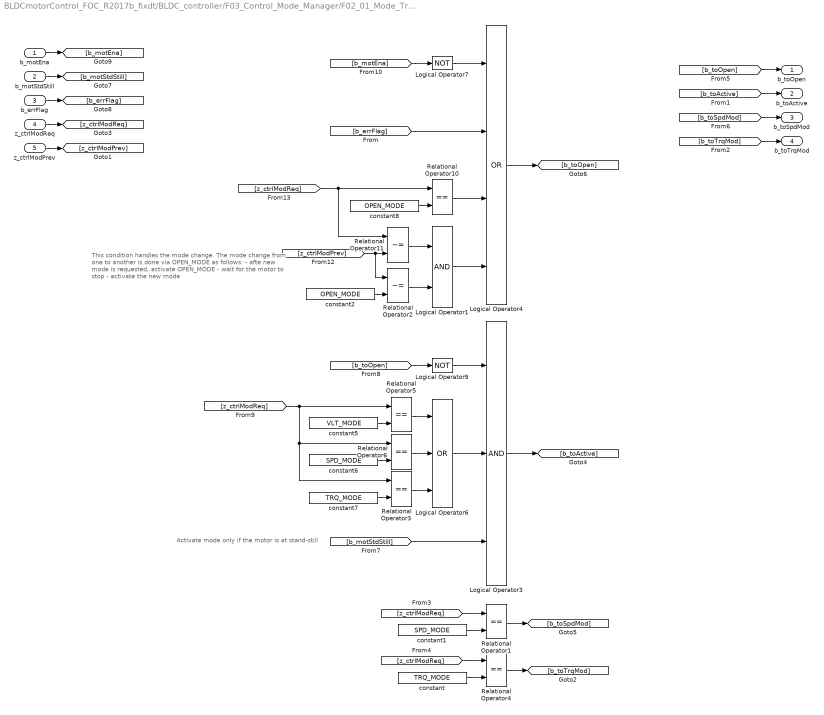
== system BLDCmotorControl_FOC_R2017b_fixdt/BLDC_controller/F03_Control_Mode_Manager/F02_01_Mode_Transition_Calculation ==
  note: This condition handles the mode change. The mode change from one to another is done via OPEN_MODE as follows:
      | - afte new mode is requested, activate OPEN_MODE
      | - wait for the motor to stop
      | - activate the new mode
  note: Activate mode only if the motor is at stand-still
  b_motEna : Inport
  b_motStdStill : Inport  Port=2
  b_errFlag : Inport  Port=3
  z_ctrlModReq : Inport  Port=4
  z_ctrlModPrev : Inport  Port=5
  Logical Operator1 : Logic  AllPortsSameDT=off  OutDataTypeStr=boolean
  Logical Operator3 : Logic  Inputs=3  AllPortsSameDT=off  OutDataTypeStr=boolean
  Logical Operator4 : Logic  Operator=OR  Inputs=4  AllPortsSameDT=off  OutDataTypeStr=boolean
  Logical Operator6 : Logic  Operator=OR  Inputs=3  AllPortsSameDT=off  OutDataTypeStr=boolean
  Logical Operator7 : Logic  Operator=NOT  AllPortsSameDT=off  OutDataTypeStr=boolean
  Logical Operator9 : Logic  Operator=NOT  AllPortsSameDT=off  OutDataTypeStr=boolean
  Relational Operator{1,3..6,10} (6 alike) : RelationalOperator  Operator===  OutDataTypeStr=boolean  RndMeth=Simplest
  Relational Operator11 : RelationalOperator  Operator=~=  OutDataTypeStr=boolean  RndMeth=Simplest
  Relational Operator2 : RelationalOperator  Operator=~=  OutDataTypeStr=boolean  RndMeth=Simplest
  constant : Constant  Value=TRQ_MODE  OutDataTypeStr=Inherit: Inherit via back propagation
  constant1 : Constant  Value=SPD_MODE  OutDataTypeStr=Inherit: Inherit via back propagation
  constant2 : Constant  Value=OPEN_MODE  OutDataTypeStr=Inherit: Inherit via back propagation
  constant5 : Constant  Value=VLT_MODE  OutDataTypeStr=Inherit: Inherit via back propagation
  constant6 : Constant  Value=SPD_MODE  OutDataTypeStr=Inherit: Inherit via back propagation
  constant7 : Constant  Value=TRQ_MODE  OutDataTypeStr=Inherit: Inherit via back propagation
  constant8 : Constant  Value=OPEN_MODE  OutDataTypeStr=Inherit: Inherit via back propagation
  b_toOpen : Outport  OutputWhenDisabled=reset  InitialOutput=0
  b_toActive : Outport  Port=2  OutputWhenDisabled=reset  InitialOutput=0
  b_toSpdMod : Outport  Port=3  OutputWhenDisabled=reset  InitialOutput=0
  b_toTrqMod : Outport  Port=4  OutputWhenDisabled=reset  InitialOutput=0
  wires:
  Relational Operator6/1 -> Logical Operator6/2
  constant6/1 -> Relational Operator6/2
  constant7/1 -> Relational Operator3/2
  Relational Operator3/1 -> Logical Operator6/3
  Relational Operator4/1 -> [b_toTrqMod]
  Logical Operator3/1 -> [b_toActive]
  [z_ctrlModReq] -> Relational Operator11/1, Relational Operator10/1
  constant5/1 -> Relational Operator5/2
  [z_ctrlModReq] -> Relational Operator4/1
  constant/1 -> Relational Operator4/2
  constant1/1 -> Relational Operator1/2
  Relational Operator1/1 -> [b_toSpdMod]
  [z_ctrlModReq] -> Relational Operator1/1
  Relational Operator5/1 -> Logical Operator6/1
  [z_ctrlModReq] -> Relational Operator6/1, Relational Operator3/1, Relational Operator5/1
  Logical Operator9/1 -> Logical Operator3/1
  constant2/1 -> Relational Operator2/2
  Relational Operator10/1 -> Logical Operator4/3
  [z_ctrlModPrev] -> Relational Operator2/1, Relational Operator11/2
  [b_motEna] -> Logical Operator7/1
  [b_toOpen] -> Logical Operator9/1
  Logical Operator4/1 -> [b_toOpen]
  Relational Operator2/1 -> Logical Operator1/2
  Relational Operator11/1 -> Logical Operator1/1
  Logical Operator6/1 -> Logical Operator3/2
  constant8/1 -> Relational Operator10/2
  Logical Operator1/1 -> Logical Operator4/4
  Logical Operator7/1 -> Logical Operator4/1
  [b_motStdStill] -> Logical Operator3/3
  b_motEna/1 -> [b_motEna]
  z_ctrlModReq/1 -> [z_ctrlModReq]
  z_ctrlModPrev/1 -> [z_ctrlModPrev]
  [b_toOpen] -> b_toOpen/1
  [b_toActive] -> b_toActive/1
  [b_toTrqMod] -> b_toTrqMod/1
  [b_toSpdMod] -> b_toSpdMod/1
  b_errFlag/1 -> [b_errFlag]
  [b_errFlag] -> Logical Operator4/2
  b_motStdStill/1 -> [b_motStdStill]

== system BLDCmotorControl_FOC_R2017b_fixdt/BLDC_controller/F04_Field_Oriented_Control/Clarke_Transform ==
  i_phaAB : Inport
  i_phaBC : Inport  Port=2
  Clarke_PhasesAB : Subsystem
  Clarke_PhasesBC : Subsystem
  If1 : If  IfExpression=u1 ~= 0
  Merge : Merge
  Merge1 : Merge
  b_selPhaABCurrMeas : Constant  Value=b_selPhaABCurrMeas  OutDataTypeStr=boolean
  i_alpha : Outport
  i_beta : Outport  Port=2
  wires:
  Clarke_PhasesBC/1(i_alphaBC) -> [i_alphaBC]
  [i_betaBC] -> Merge1/2
  [i_betaAB] -> Merge1/1
  i_phaAB/1 -> [i_phaAB]
  [i_phaBC] -> Clarke_PhasesBC/2(i_phaC)
  [i_phaAB] -> Clarke_PhasesBC/1(i_phaB)
  Clarke_PhasesAB/1(i_alphaAB) -> [i_alphaAB]
  [i_alphaAB] -> Merge/1
  If1/1 -> Clarke_PhasesAB/Action
  b_selPhaABCurrMeas/1 -> If1/1
  If1/2 -> Clarke_PhasesBC/Action
  [i_alphaBC] -> Merge/2
  [i_beta] -> i_beta/1
  Clarke_PhasesAB/2(i_betaAB) -> [i_betaAB]
  i_phaBC/1 -> [i_phaBC]
  [i_phaBC] -> Clarke_PhasesAB/2(i_phaB)
  Merge1/1 -> [i_beta]
  Merge/1 -> [i_alpha]
  [i_phaAB] -> Clarke_PhasesAB/1(i_phaA)
  [i_alpha] -> i_alpha/1
  Clarke_PhasesBC/2(i_betaBC) -> [i_betaBC]

== system BLDCmotorControl_FOC_R2017b_fixdt/BLDC_controller/F04_Field_Oriented_Control/Current_Filtering ==
  iq_raw : Inport
  id_raw : Inport  Port=2
  Demux1 : Demux  Outputs=2
  Low_Pass_Filter : BLDC_controller_Lib/Low_Pass_Filter  SystemSampleTime=-1
  Mux2 : Mux  Inputs=2
  cf_currFilt : Constant  Value=cf_currFilt  OutDataTypeStr=fixdt(0,16,16)
  iq : Outport
  id : Outport  Port=2
  wires:
  Mux2/1 -> Low_Pass_Filter/1
  Demux1/2 -> [id]
  cf_currFilt/1 -> Low_Pass_Filter/2
  id_raw/1 -> [id_raw]
  [iq] -> iq/1
  [id] -> id/1
  iq_raw/1 -> [iq_raw]
  Demux1/1 -> [iq]
  Low_Pass_Filter/1 -> Demux1/1
  [iq_raw] -> Mux2/1
  [id_raw] -> Mux2/2

== system BLDCmotorControl_FOC_R2017b_fixdt/BLDC_controller/F04_Field_Oriented_Control/Field_Weakening ==
  note: Sine/Cosine Look-up Tables
  note: FOC Field weakening
  note: Note: The Sine and Cosine maps are shifted in phase by 30 deg to align with the Hall sensors position.
  note: Field Weakening map as a function of Motor Speed
  a_elecAngle : Inport
  n_motAbs : Inport  Port=2
  Data Type Conversion : DataTypeConversion  OutDataTypeStr=fixdt(1,16,4)
  Switch1 : Switch  Criteria=u2 ~= 0  OutDataTypeStr=Inherit: Inherit via back propagation  RndMeth=Zero
  a_elecAngle_XA : PreLookup  BreakpointsData=a_elecAngle_XA  OutputSelection=Index only  IndexSearchMethod=Evenly spaced points  BeginIndexSearchUsingPreviousIndexResult=on  IndexDataTypeStr=uint8  FractionDataTypeStr=fixdt(0,16,14)  RndMeth=Simplest
  a_elecPeriod1 : Constant  Value=0  OutDataTypeStr=Inherit: Inherit via back propagation
  a_elecPeriod3 : Constant  Value=0  OutDataTypeStr=uint8
  b_fieldWeakEna : Constant  Value=b_fieldWeakEna  OutDataTypeStr=boolean
  id_fieldWeak_M1 : Interpolation_n-D  NumberOfTableDimensions=1  Table=id_fieldWeak_M1  ExtrapMethod=Clip  OutDataTypeStr=fixdt(0,10,0)  InternalRulePriority=Speed  RndMeth=Simplest
      settings: InputPortMap=u0,u1
  n_fieldWeak_XA : PreLookup  BreakpointsData=n_fieldWeak_XA  IndexSearchMethod=Evenly spaced points  BeginIndexSearchUsingPreviousIndexResult=on  IndexDataTypeStr=uint8  FractionDataTypeStr=fixdt(0,8,6)  RndMeth=Simplest
  r_cos_M1 : Interpolation_n-D  NumberOfTableDimensions=1  Table=r_cos_M1  InterpMethod=Flat  ExtrapMethod=Clip  ValidIndexMayReachLast=on  OutDataTypeStr=fixdt(1,16,14)  InternalRulePriority=Speed  RndMeth=Simplest
      settings: InputPortMap=u0,u1
  r_sin_M1 : Interpolation_n-D  NumberOfTableDimensions=1  Table=r_sin_M1  InterpMethod=Flat  ExtrapMethod=Clip  ValidIndexMayReachLast=on  OutDataTypeStr=fixdt(1,16,14)  InternalRulePriority=Speed  RndMeth=Simplest
      settings: InputPortMap=u0,u1
  toNegative : Gain  Tag=struct('comment',struct('text','','placement',1),'logdata',struct('maxnumvals',inf,'plotchannels',[],'loggingmode',3,'channels',1),'output',struct('variable','','description','','name','$S_$B','width',1,'address','','max',NaN,'min',NaN,'class','default','type','CONTINUOUS','scaling','','lsb',1,'offset',0,'arb',0,'freeze',1,'unit','','autoscalingmode',1,'lowerheadroom',1,'upperheadroom',1,'headroomunit','bit','keepdatatype',1,'checkmin',0,'checkmax',0,'castoutput',0,'show',0),'gain',struct('variable','','description','','name','$S_$B_gain','width',1,'address','','max',NaN,'min',NaN,'class','default','type','CONTINUOUS','scaling','','lsb',1,'offset',0,'arb',0,'freeze',1,'unit','','keepdatatype',1,'value','1','scalar',0,'tolerance',1),'scalingvalid',0,'date',730486)  Gain=-1  OutDataTypeStr=fixdt(1,16,4)  RndMeth=Zero  ParamDataTypeStr=Inherit: Same as input
  r_sin : Outport
  r_cos : Outport  Port=2
  id_Tgt : Outport  Port=3
  id_TgtAbs : Outport  Port=4
  wires:
  a_elecAngle_XA/1 -> r_cos_M1/1, r_sin_M1/1
  r_sin_M1/1 -> r_sin/1
  a_elecAngle/1 -> a_elecAngle_XA/1
  r_cos_M1/1 -> r_cos/1
  a_elecPeriod3/1 -> r_cos_M1/2, r_sin_M1/2
  n_fieldWeak_XA/1 -> id_fieldWeak_M1/1
  id_fieldWeak_M1/1 -> Data Type Conversion/1
  n_fieldWeak_XA/2 -> id_fieldWeak_M1/2
  b_fieldWeakEna/1 -> Switch1/2
  Data Type Conversion/1 -> Switch1/1
  a_elecPeriod1/1 -> Switch1/3
  n_motAbs/1 -> n_fieldWeak_XA/1
  toNegative/1 -> id_Tgt/1
  Switch1/1 -> id_TgtAbs/1, toNegative/1

== system BLDCmotorControl_FOC_R2017b_fixdt/BLDC_controller/F04_Field_Oriented_Control/Inv_Clarke_Transform ==
  note: Inverse Clarke Transform:
      | V_phaA = V_alpha
      | V_phaB = -(1/2)*V_alpha + (sqrt(3)/2)*V_beta
      | V_phaC = -VphaA - V_phaB
  note: Space Vector Modulation (SVM)
  V_alpha : Inport
  V_beta : Inport  Port=2
  Add : Sum  SaturateOnIntegerOverflow=on
  Add1 : Sum  Inputs=-+  SaturateOnIntegerOverflow=on  OutDataTypeStr=Inherit: Same as first input
  Demux : Demux  Outputs=3
  Gain1 : Gain  Tag=struct('comment',struct('text','','placement',1),'logdata',struct('maxnumvals',inf,'plotchannels',[],'loggingmode',3,'channels',1),'output',struct('variable','','description','','name','$S_$B','width',1,'address','','max',NaN,'min',NaN,'class','default','type','CONTINUOUS','scaling','','lsb',1,'offset',0,'arb',0,'freeze',1,'unit','','autoscalingmode',1,'lowerheadroom',1,'upperheadroom',1,'headroomunit','bit','keepdatatype',1,'checkmin',0,'checkmax',0,'castoutput',0,'show',0),'gain',struct('variable','','description','','name','$S_$B_gain','width',1,'address','','max',NaN,'min',NaN,'class','default','type','CONTINUOUS','scaling','','lsb',1,'offset',0,'arb',0,'freeze',1,'unit','','keepdatatype',1,'value','1','scalar',0,'tolerance',1),'scalingvalid',0,'date',730486)  Gain=sqrt(3)/2  OutDataTypeStr=fixdt(1,16,5)  RndMeth=Zero
  Gain2 : Gain  Gain=0.5  OutDataTypeStr=Inherit: Same as input
  Gain3 : Gain  Tag=struct('comment',struct('text','','placement',1),'logdata',struct('maxnumvals',inf,'plotchannels',[],'loggingmode',3,'channels',1),'output',struct('variable','','description','','name','$S_$B','width',1,'address','','max',NaN,'min',NaN,'class','default','type','CONTINUOUS','scaling','','lsb',1,'offset',0,'arb',0,'freeze',1,'unit','','autoscalingmode',1,'lowerheadroom',1,'upperheadroom',1,'headroomunit','bit','keepdatatype',1,'checkmin',0,'checkmax',0,'castoutput',0,'show',0),'gain',struct('variable','','description','','name','$S_$B_gain','width',1,'address','','max',NaN,'min',NaN,'class','default','type','CONTINUOUS','scaling','','lsb',1,'offset',0,'arb',0,'freeze',1,'unit','','keepdatatype',1,'value','1','scalar',0,'tolerance',1),'scalingvalid',0,'date',730486)  Gain=1/2  OutDataTypeStr=fixdt(1,16,5)  RndMeth=Zero
  Gain4 : Gain  Gain=2/sqrt(3)  OutDataTypeStr=fixdt(1,16,0)
  MinMax1 : MinMax  InputSameDT=on
  MinMax2 : MinMax  Function=max  InputSameDT=on
  Mux4 : Mux  Inputs=3
  Sum2 : Sum  Inputs=--  OutDataTypeStr=fixdt(1,16,4)  RndMeth=Simplest  SaturateOnIntegerOverflow=on
  Sum6 : Sum  Inputs=-+  OutDataTypeStr=fixdt(1,16,4)  RndMeth=Simplest  SaturateOnIntegerOverflow=on
  V_phaA : Outport
  V_phaB : Outport  Port=2
  V_phaC : Outport  Port=3
  wires:
  Sum6/1 -> Sum2/2, Mux4/2
  Sum2/1 -> Mux4/3
  Gain1/1 -> Sum6/2
  Gain3/1 -> Sum6/1
  V_alpha/1 -> Gain3/1, Sum2/1, Mux4/1  "alpha"
  V_beta/1 -> Gain1/1  "beta"
  Add/1 -> Gain2/1
  Add1/1 -> Gain4/1
  MinMax1/1 -> Add/1
  Demux/3 -> V_phaC/1
  Demux/2 -> V_phaB/1
  Gain2/1 -> Add1/1
  Demux/1 -> V_phaA/1
  MinMax2/1 -> Add/2
  Mux4/1 -> Add1/2, MinMax2/1, MinMax1/1
  Gain4/1 -> Demux/1

== system BLDCmotorControl_FOC_R2017b_fixdt/BLDC_controller/F04_Field_Oriented_Control/Inv_Park_Transform ==
  note: Inverse Park Transform:
      | V_alpha = Vd*cos(angle) - Vq*sin(angle)
      | V_beta = Vd*sin(angle) + Vq*cos(angle)
  Vq : Inport
  Vd : Inport  Port=2
  r_sin : Inport  Port=3
  r_cos : Inport  Port=4
  Divide{1..4} (4 alike) : Product  Inputs=**  OutDataTypeStr=fixdt(1,16,5)  RndMeth=Simplest
  Sum1 : Sum  OutDataTypeStr=fixdt(1,16,4)  RndMeth=Simplest  SaturateOnIntegerOverflow=on
  Sum6 : Sum  Inputs=+-  OutDataTypeStr=fixdt(1,16,4)  RndMeth=Simplest  SaturateOnIntegerOverflow=on
  V_alpha : Outport
  V_beta : Outport  Port=2
  wires:
  r_sin/1 -> [r_sin]
  Vd/1 -> [Vd]
  Vq/1 -> [Vq]
  r_cos/1 -> [r_cos]
  [r_cos] -> Divide4/2
  [r_sin] -> Divide1/2
  [Vd] -> Divide4/1
  [r_cos] -> Divide3/2
  Divide1/1 -> Sum6/2
  [Vq] -> Divide1/1
  [Vd] -> Divide2/1
  Divide2/1 -> Sum1/1
  Divide3/1 -> Sum1/2
  [Vq] -> Divide3/1
  Divide4/1 -> Sum6/1
  [r_sin] -> Divide2/2
  Sum1/1 -> V_beta/1
  Sum6/1 -> V_alpha/1
